simulink model "quadcopter"  (R2023a)
settings: Solver=VariableStepAuto  StartTime=0.0  StopTime=inf  RelTol=1e-3
libraries: slpidlib x4, simulink x1, vrlib x1
settings Model: Creator=sait karadeniz  LastModifiedBy=sait karadeniz
settings DataIOCC: ReturnWorkspaceOutputs=off

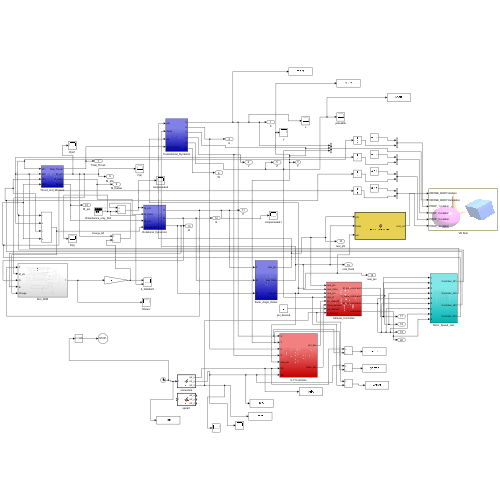
[thumbnail: Simulink's stored preview of the top-level diagram]
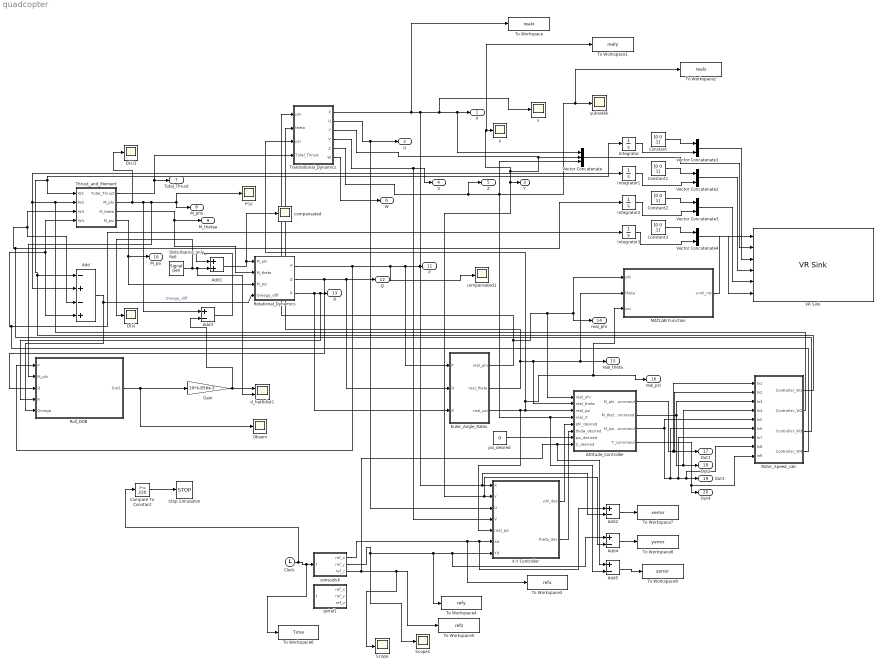
== system quadcopter ==
  Add : Sum  Inputs=-+-+
  Add1 : Sum
  Add{2..5} (4 alike) : Sum  Inputs=+-
  Attitude_Controller : Subsystem
  Clock : Clock
  Compare To Constant : simulink/Logic and Bit Operations/Compare To Constant  relop=>=  const=220  OutDataTypeStr=boolean
  Constant{,1..3} (4 alike) : Constant  Value=[0 0 1]  OutMax=[3]
  D(s) : Scope
  D(s)1 : Scope
  "Disturbance_only_Roll " : SignalGenerator  Amplitude=0.0  Frequency=2  Units=rad/sec
  Euler_Angle_Rates : Subsystem
  F(s) : Scope
  Gain : Gain  Gain=10*4.856e-3
  Integrator{,1..3} (4 alike) : Integrator
  MATLAB Function : MATLAB Function  TreatAsAtomicUnit=on
  Observ : Scope
  Roll_DOB : Subsystem
  Rotational_Dynamics : Subsystem
  Rotor_Speed_calc : Subsystem
  Scope : Scope
  Scope1 : Scope
  Stop Simulation : Stop
  Thrust_and_Moment : Subsystem
  To Workspace : ToWorkspace  VariableName=realx  SampleTime=-1
  To Workspace1 : ToWorkspace  VariableName=realy  SampleTime=-1
  To Workspace2 : ToWorkspace  VariableName=realz  SampleTime=-1
  To Workspace3 : ToWorkspace  VariableName=refx  SampleTime=-1
  To Workspace4 : ToWorkspace  VariableName=refy  SampleTime=-1
  To Workspace5 : ToWorkspace  VariableName=refz  SampleTime=-1
  To Workspace6 : ToWorkspace  VariableName=Time  SampleTime=-1
  To Workspace7 : ToWorkspace  VariableName=xerror  SampleTime=-1
  To Workspace8 : ToWorkspace  VariableName=yerror  SampleTime=-1
  To Workspace9 : ToWorkspace  VariableName=zerror  SampleTime=-1
  Translational_Dynamics : Subsystem
  VR Sink : vrlib/VR Sink  InstantiateOnLoad=on  SampleTime=0.1  ViewEnable=on  RemoteChange=off  RemoteView=off  FieldsWritten=DRONE_BODY.rotation.4.1.1.double#DRONE_BODY.translation.3.1.1.double#PROP_1.rotation.4.1.1.double#PROP_2.rotation.4.1.1.double#PROP_3.rotation.4.1.1.double#PROP_4.rotation.4.1.1.double  WorldFileName=C:\Documents\quadcopter.wrl  WorldDescription=Quadcopter World  AutoView=on  VideoDimensions=[]  AllowVariableSize=off
  Vector Concatenate : Concatenate  NumInputs=3
  Vector Concatenate{1..4} (4 alike) : Concatenate
  X-Y Controller : Subsystem
  compansated : Scope
  compansated1 : Scope
  d_hat6dist1 : Scope  NumInputPorts=2
  psi_desired : Constant  Value=0
  sonsuzluk : MATLAB Function  TreatAsAtomicUnit=on
  spiral1 : MATLAB Function  TreatAsAtomicUnit=on
  x : Scope
  y : Scope
  yükseklik : Scope
  X : Outport
  U : Outport  Port=2
  Y : Outport  Port=3
  V : Outport  Port=4
  Z : Outport  Port=5
  W : Outport  Port=6
  Total_Thrust : Outport  Port=7
  M_phii : Outport  Port=8
  M_thetaa : Outport  Port=9
  M_psi : Outport  Port=10
  P : Outport  Port=11
  Q : Outport  Port=12
  R : Outport  Port=13
  real_phi : Outport  Port=14
  real_theta : Outport  Port=15
  real_psi : Outport  Port=16
  Out1 : Outport  Port=17
  Out2 : Outport  Port=18
  Out3 : Outport  Port=19
  Out4 : Outport  Port=20
  wires:
  Thrust_and_Moment/1(Total_Thrust) -> Translational_Dynamics/4(Total_Thrust), Total_Thrust/1
  Thrust_and_Moment/2(M_phi) -> D(s)1/1, F(s)/1, M_phii/1, Roll_DOB/2(M_phi), Add3/1
  Thrust_and_Moment/3(M_theta) -> Rotational_Dynamics/2(M_theta), M_thetaa/1
  Euler_Angle_Rates/1(real_phi) -> Translational_Dynamics/1(phi), Attitude_Controller/1(real_phi), MATLAB Function/1(phi), real_phi/1
  Euler_Angle_Rates/3(real_psi) -> Attitude_Controller/3(real_psi), Translational_Dynamics/3(psi), real_psi/1, MATLAB Function/3(psi), X-Y Controller/5(real_psi)
  Translational_Dynamics/1(X) -> To Workspace/1, x/1, Vector Concatenate/1, X/1, Add2/2, X-Y Controller/1(X)
  Translational_Dynamics/2(U) -> X-Y Controller/3(U), U/1
  Translational_Dynamics/3(Y) -> Add4/2, X-Y Controller/2(Y), Y/1, To Workspace1/1, y/1, Vector Concatenate/2
  Translational_Dynamics/4(V) -> X-Y Controller/4(V), V/1
  Translational_Dynamics/5(Z) -> To Workspace2/1, yükseklik/1, Add5/2, Attitude_Controller/4(real_Z), Vector Concatenate/3, Z/1
  Translational_Dynamics/6(W) -> W/1
  Add/1 -> Roll_DOB/5(Omega), Rotational_Dynamics/4(Omega_diff)  "Omega_diff"
  Rotational_Dynamics/2(Q) -> Euler_Angle_Rates/2(Q), Q/1, Roll_DOB/3(Q)
  Rotational_Dynamics/3(R) -> Euler_Angle_Rates/3(R), Roll_DOB/4(R), R/1
  Rotational_Dynamics/1(P) -> Roll_DOB/1(P), compansated1/1, Euler_Angle_Rates/1(P), P/1
  Rotor_Speed_calc/1(Controller_W1) -> Integrator/1, Thrust_and_Moment/1(W1), Add/1
  Rotor_Speed_calc/2(Controller_W2) -> Add/2, Integrator1/1, Thrust_and_Moment/2(W2)
  Rotor_Speed_calc/3(Controller_W3) -> Thrust_and_Moment/3(W3), Add/3, Integrator2/1
  Rotor_Speed_calc/4(Controller_W4) -> Add/4, Thrust_and_Moment/4(W4), Integrator3/1
  Vector Concatenate/1 -> VR Sink/2
  MATLAB Function/1(vrml_rot) -> VR Sink/1
  Constant/1 -> Vector Concatenate1/1
  Integrator/1 -> Vector Concatenate1/2
  Constant1/1 -> Vector Concatenate2/1
  Integrator1/1 -> Vector Concatenate2/2
  Constant2/1 -> Vector Concatenate3/1
  Integrator2/1 -> Vector Concatenate3/2
  Constant3/1 -> Vector Concatenate4/1
  Integrator3/1 -> Vector Concatenate4/2
  Vector Concatenate1/1 -> VR Sink/3
  Vector Concatenate2/1 -> VR Sink/4
  Vector Concatenate3/1 -> VR Sink/5
  Vector Concatenate4/1 -> VR Sink/6
  Euler_Angle_Rates/2(real_theta) -> Translational_Dynamics/2(theta), Attitude_Controller/2(real_theta), MATLAB Function/2(theta), real_theta/1
  Attitude_Controller/1(M_phi_command) -> Rotor_Speed_calc/1(In1), Rotor_Speed_calc/2(In2), Out1/1
  Attitude_Controller/2(M_theta_command) -> Rotor_Speed_calc/4(In4), Out2/1, Rotor_Speed_calc/3(In3)
  Attitude_Controller/3(M_psi_command) -> Rotor_Speed_calc/6(In6), Rotor_Speed_calc/7(In7), Rotor_Speed_calc/8(In8), Out3/1, Rotor_Speed_calc/5(In5)
  Attitude_Controller/4(T_command) -> Out4/1, Rotor_Speed_calc/9(In9)
  Add1/1 -> compansated/1, Rotational_Dynamics/1(M_phi)
  Thrust_and_Moment/4(M_psi) -> Rotational_Dynamics/3(M_psi), M_psi/1
  psi_desired/1 -> Attitude_Controller/7(psi_desired)
  X-Y Controller/1(phi_des) -> Attitude_Controller/5(phi_desired)
  X-Y Controller/2(theta_des) -> Attitude_Controller/6(theta_desired)
  Add3/1 -> Add1/1
  "Disturbance_only_Roll "/1 -> D(s)/1, d_hat6dist1/2, Add1/2
  Roll_DOB/1(Out1) -> Gain/1, Observ/1
  Gain/1 -> Add3/2, d_hat6dist1/1
  Clock/1 -> Compare To Constant/1, To Workspace6/1, sonsuzluk/1(t)
  sonsuzluk/1(ref_x) -> To Workspace3/1, Add2/1, X-Y Controller/6(Xd)
  sonsuzluk/3(ref_z) -> Scope/1, To Workspace5/1, Add5/1, Attitude_Controller/8(Z_desired)
  sonsuzluk/2(ref_y) -> Scope1/1, Add4/1, X-Y Controller/7(Yd), To Workspace4/1
  Compare To Constant/1 -> Stop Simulation/1
  Add2/1 -> To Workspace7/1
  Add4/1 -> To Workspace8/1
  Add5/1 -> To Workspace9/1

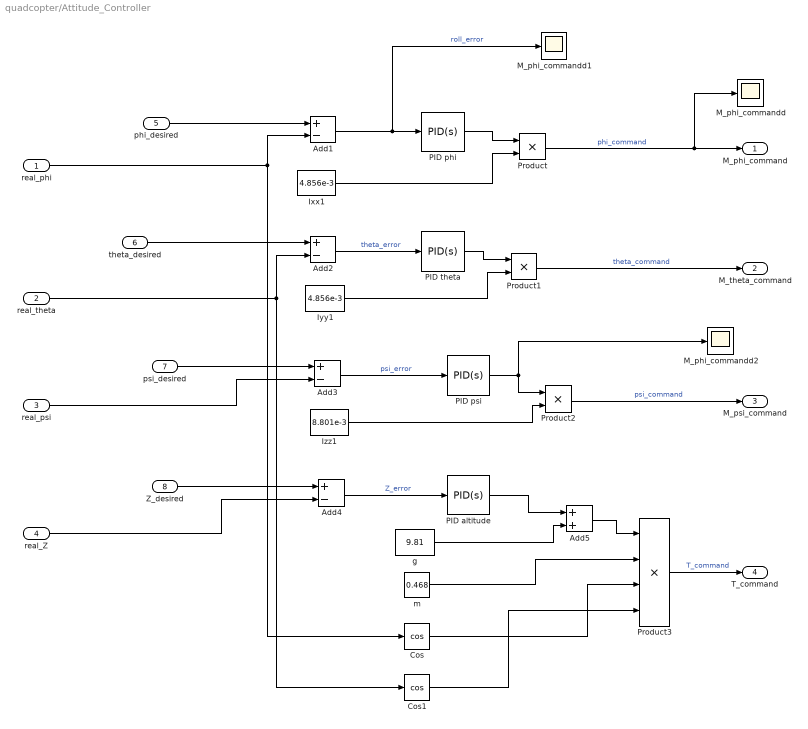
== system quadcopter/Attitude_Controller ==
  real_phi : Inport
  real_theta : Inport  Port=2
  real_psi : Inport  Port=3
  real_Z : Inport  Port=4
  phi_desired : Inport  Port=5
  theta_desired : Inport  Port=6
  psi_desired : Inport  Port=7
  Z_desired : Inport  Port=8
  Add{1..4} (4 alike) : Sum  Inputs=+-
  Add5 : Sum
  Cos : Trigonometry  Operator=cos
  Cos1 : Trigonometry  Operator=cos
  Ixx1 : Constant  Value=4.856e-3
  Iyy1 : Constant  Value=4.856e-3
  Izz1 : Constant  Value=8.801e-3
  M_phi_commandd : Scope
  M_phi_commandd1 : Scope
  M_phi_commandd2 : Scope
  PID altitude : slpidlib/PID Controller  Controller=PID  Form=Parallel  TimeDomain=Continuous-time  UseExternalTs=off  SampleTime=-1  IntegratorMethod=Forward Euler  FilterMethod=Forward Euler  ControllerParametersSource=internal  P=0.3437  I=0.0034  UseKiTs=off  D=0.5550  N=100  UseFilter=on  TunerSelectOption=Transfer Function Based (PID Tuner App)  InitialConditionSource=internal  InitialConditionForIntegrator=0  InitialConditionForFilter=0  DifferentiatorICPrevScaledInput=0  ExternalReset=none  TrackingMode=off  Kt=1  LimitOutput=off  SatLimitsSource=internal  UpperSaturationLimit=inf  LowerSaturationLimit=-inf  LinearizeAsGain=on  AntiWindupMode=none  Kb=1  LimitIntegrator=off  UpperIntegratorSaturationLimit=inf  LowerIntegratorSaturationLimit=-inf  POutMin=[]  POutMax=[]  IOutMin=[]  IOutMax=[]  DOutMin=[]  DOutMax=[]  NOutMin=[]  NOutMax=[]  SumOutMin=[]  SumOutMax=[]  SaturationOutMin=[]  SaturationOutMax=[]  PParamMin=[]  PParamMax=[]  IParamMin=[]  IParamMax=[]  DParamMin=[]  DParamMax=[]  NParamMin=[]  NParamMax=[]  KbParamMin=[]  KbParamMax=[]  KtParamMin=[]  KtParamMax=[]  KbOutMin=[]  KbOutMax=[]  KtOutMin=[]  KtOutMax=[]  IntegratorOutMin=[]  IntegratorOutMax=[]  FilterOutMin=[]  FilterOutMax=[]  SumI1OutMin=[]  SumI1OutMax=[]  SumI2OutMin=[]  SumI2OutMax=[]  SumI3OutMin=[]  SumI3OutMax=[]  SumI4OutMin=[]  SumI4OutMax=[]  SumDOutMin=[]  SumDOutMax=[]  DifferentiatorOutMin=[]  DifferentiatorOutMax=[]  FilterDiffOutCoefMin=[]  FilterDiffOutCoefMax=[]  ReciprocalOutMin=[]  ReciprocalOutMax=[]  SumDenOutMin=[]  SumDenOutMax=[]  SumNumOutMin=[]  SumNumOutMax=[]  DivideOutMin=[]  DivideOutMax=[]  UdiffTsProdOutMin=[]  UdiffTsProdOutMax=[]  NTsProdOutMin=[]  NTsProdOutMax=[]  UintegralTsProdOutMin=[]  UintegralTsProdOutMax=[]  UngainTsProdOutMin=[]  UngainTsProdOutMax=[]  ClampingZeroOutDataTypeStr=Inherit: Inherit via back propagation  ClampingZeroOutMin=[]  ClampingZeroOutMax=[]  FilterDenConstantOutDataTypeStr=Inherit: Inherit via back propagation  FilterDenConstantOutMin=[]  FilterDenConstantOutMax=[]  PCopyOutDataTypeStr=Inherit: Inherit via back propagation  PCopyOutMin=[]  PCopyOutMax=[]  NCopyOutDataTypeStr=Inherit: Inherit via back propagation  NCopyOutMin=[]  NCopyOutMax=[]  IntegratorContinuousStateAttributes=''  IntegratorStateMustResolveToSignalObject=off  IntegratorRTWStateStorageClass=Auto  FilterContinuousStateAttributes=''  FilterStateMustResolveToSignalObject=off  FilterRTWStateStorageClass=Auto  ParallelPVariant=InternalParameters  IdealPVariant=Disabled  IVariant=InternalParameters  DVariant=InternalParameters  IntegratorVariant=Continuous  SatVariant=Disabled  AWVariant=Passthrough  PCopyVariant=Disabled  TRVariant=Disabled  FdbkBlocksVariant=Forward  IdealPFdbkVariant=Disabled  SatFdbkVariant=Disabled  DerivativeFilterVariant=ContFilter  NVariant=InternalParameters  NCopyVariant=Disabled  FilterICVariant=InternalICsFilter  IntegratorICVariant=InternalICs  ExternalResetVariant=Disabled  TRSumVariant=Passthrough  SumFdbkVariant=Disabled  SumVariant=Sum_PID  TsampFilterVariant=InternalTs  TsampNgainVariant=Passthrough  TsampIntegralVariant=Disabled_SignalSpec  ExternalSaturationOutDataTypeStr=Inherit: Same as second input
  PID phi : slpidlib/PID Controller  Controller=PID  Form=Parallel  TimeDomain=Continuous-time  UseExternalTs=off  SampleTime=-1  IntegratorMethod=Forward Euler  FilterMethod=Forward Euler  ControllerParametersSource=internal  P=6  I=1.5  UseKiTs=off  D=2  N=20  UseFilter=on  TunerSelectOption=Transfer Function Based (PID Tuner App)  InitialConditionSource=internal  InitialConditionForIntegrator=0  InitialConditionForFilter=0  DifferentiatorICPrevScaledInput=0  ExternalReset=none  TrackingMode=off  Kt=1  LimitOutput=off  SatLimitsSource=internal  UpperSaturationLimit=inf  LowerSaturationLimit=-inf  LinearizeAsGain=on  AntiWindupMode=none  Kb=1  LimitIntegrator=off  UpperIntegratorSaturationLimit=inf  LowerIntegratorSaturationLimit=-inf  POutMin=[]  POutMax=[]  IOutMin=[]  IOutMax=[]  DOutMin=[]  DOutMax=[]  NOutMin=[]  NOutMax=[]  SumOutMin=[]  SumOutMax=[]  SaturationOutMin=[]  SaturationOutMax=[]  PParamMin=[]  PParamMax=[]  IParamMin=[]  IParamMax=[]  DParamMin=[]  DParamMax=[]  NParamMin=[]  NParamMax=[]  KbParamMin=[]  KbParamMax=[]  KtParamMin=[]  KtParamMax=[]  KbOutMin=[]  KbOutMax=[]  KtOutMin=[]  KtOutMax=[]  IntegratorOutMin=[]  IntegratorOutMax=[]  FilterOutMin=[]  FilterOutMax=[]  SumI1OutMin=[]  SumI1OutMax=[]  SumI2OutMin=[]  SumI2OutMax=[]  SumI3OutMin=[]  SumI3OutMax=[]  SumI4OutMin=[]  SumI4OutMax=[]  SumDOutMin=[]  SumDOutMax=[]  DifferentiatorOutMin=[]  DifferentiatorOutMax=[]  FilterDiffOutCoefMin=[]  FilterDiffOutCoefMax=[]  ReciprocalOutMin=[]  ReciprocalOutMax=[]  SumDenOutMin=[]  SumDenOutMax=[]  SumNumOutMin=[]  SumNumOutMax=[]  DivideOutMin=[]  DivideOutMax=[]  UdiffTsProdOutMin=[]  UdiffTsProdOutMax=[]  NTsProdOutMin=[]  NTsProdOutMax=[]  UintegralTsProdOutMin=[]  UintegralTsProdOutMax=[]  UngainTsProdOutMin=[]  UngainTsProdOutMax=[]  ClampingZeroOutDataTypeStr=Inherit: Inherit via back propagation  ClampingZeroOutMin=[]  ClampingZeroOutMax=[]  FilterDenConstantOutDataTypeStr=Inherit: Inherit via back propagation  FilterDenConstantOutMin=[]  FilterDenConstantOutMax=[]  PCopyOutDataTypeStr=Inherit: Inherit via back propagation  PCopyOutMin=[]  PCopyOutMax=[]  NCopyOutDataTypeStr=Inherit: Inherit via back propagation  NCopyOutMin=[]  NCopyOutMax=[]  IntegratorContinuousStateAttributes=''  IntegratorStateMustResolveToSignalObject=off  IntegratorRTWStateStorageClass=Auto  FilterContinuousStateAttributes=''  FilterStateMustResolveToSignalObject=off  FilterRTWStateStorageClass=Auto  ParallelPVariant=InternalParameters  IdealPVariant=Disabled  IVariant=InternalParameters  DVariant=InternalParameters  IntegratorVariant=Continuous  SatVariant=Disabled  AWVariant=Passthrough  PCopyVariant=Disabled  TRVariant=Disabled  FdbkBlocksVariant=Forward  IdealPFdbkVariant=Disabled  SatFdbkVariant=Disabled  DerivativeFilterVariant=ContFilter  NVariant=InternalParameters  NCopyVariant=Disabled  FilterICVariant=InternalICsFilter  IntegratorICVariant=InternalICs  ExternalResetVariant=Disabled  TRSumVariant=Passthrough  SumFdbkVariant=Disabled  SumVariant=Sum_PID  TsampFilterVariant=InternalTs  TsampNgainVariant=Passthrough  TsampIntegralVariant=Disabled_SignalSpec  ExternalSaturationOutDataTypeStr=Inherit: Same as second input
  PID psi : slpidlib/PID Controller  Controller=PID  Form=Parallel  TimeDomain=Continuous-time  UseExternalTs=off  SampleTime=-1  IntegratorMethod=Forward Euler  FilterMethod=Forward Euler  ControllerParametersSource=internal  P=0.3  I=0.001  UseKiTs=off  D=0.7  N=100  UseFilter=on  TunerSelectOption=Transfer Function Based (PID Tuner App)  InitialConditionSource=internal  InitialConditionForIntegrator=0  InitialConditionForFilter=0  DifferentiatorICPrevScaledInput=0  ExternalReset=none  TrackingMode=off  Kt=1  LimitOutput=off  SatLimitsSource=internal  UpperSaturationLimit=inf  LowerSaturationLimit=-inf  LinearizeAsGain=on  AntiWindupMode=none  Kb=1  LimitIntegrator=on  UpperIntegratorSaturationLimit=0.5  LowerIntegratorSaturationLimit=-0.5  POutMin=[]  POutMax=[]  IOutMin=[]  IOutMax=[]  DOutMin=[]  DOutMax=[]  NOutMin=[]  NOutMax=[]  SumOutMin=[]  SumOutMax=[]  SaturationOutMin=[]  SaturationOutMax=[]  PParamMin=[]  PParamMax=[]  IParamMin=[]  IParamMax=[]  DParamMin=[]  DParamMax=[]  NParamMin=[]  NParamMax=[]  KbParamMin=[]  KbParamMax=[]  KtParamMin=[]  KtParamMax=[]  KbOutMin=[]  KbOutMax=[]  KtOutMin=[]  KtOutMax=[]  IntegratorOutMin=[]  IntegratorOutMax=[]  FilterOutMin=[]  FilterOutMax=[]  SumI1OutMin=[]  SumI1OutMax=[]  SumI2OutMin=[]  SumI2OutMax=[]  SumI3OutMin=[]  SumI3OutMax=[]  SumI4OutMin=[]  SumI4OutMax=[]  SumDOutMin=[]  SumDOutMax=[]  DifferentiatorOutMin=[]  DifferentiatorOutMax=[]  FilterDiffOutCoefMin=[]  FilterDiffOutCoefMax=[]  ReciprocalOutMin=[]  ReciprocalOutMax=[]  SumDenOutMin=[]  SumDenOutMax=[]  SumNumOutMin=[]  SumNumOutMax=[]  DivideOutMin=[]  DivideOutMax=[]  UdiffTsProdOutMin=[]  UdiffTsProdOutMax=[]  NTsProdOutMin=[]  NTsProdOutMax=[]  UintegralTsProdOutMin=[]  UintegralTsProdOutMax=[]  UngainTsProdOutMin=[]  UngainTsProdOutMax=[]  ClampingZeroOutDataTypeStr=Inherit: Inherit via back propagation  ClampingZeroOutMin=[]  ClampingZeroOutMax=[]  FilterDenConstantOutDataTypeStr=Inherit: Inherit via back propagation  FilterDenConstantOutMin=[]  FilterDenConstantOutMax=[]  PCopyOutDataTypeStr=Inherit: Inherit via back propagation  PCopyOutMin=[]  PCopyOutMax=[]  NCopyOutDataTypeStr=Inherit: Inherit via back propagation  NCopyOutMin=[]  NCopyOutMax=[]  IntegratorContinuousStateAttributes=''  IntegratorStateMustResolveToSignalObject=off  IntegratorRTWStateStorageClass=Auto  FilterContinuousStateAttributes=''  FilterStateMustResolveToSignalObject=off  FilterRTWStateStorageClass=Auto  ParallelPVariant=InternalParameters  IdealPVariant=Disabled  IVariant=InternalParameters  DVariant=InternalParameters  IntegratorVariant=Continuous  SatVariant=Disabled  AWVariant=Passthrough  PCopyVariant=Disabled  TRVariant=Disabled  FdbkBlocksVariant=Forward  IdealPFdbkVariant=Disabled  SatFdbkVariant=Disabled  DerivativeFilterVariant=ContFilter  NVariant=InternalParameters  NCopyVariant=Disabled  FilterICVariant=InternalICsFilter  IntegratorICVariant=InternalICs  ExternalResetVariant=Disabled  TRSumVariant=Passthrough  SumFdbkVariant=Disabled  SumVariant=Sum_PID  TsampFilterVariant=InternalTs  TsampNgainVariant=Passthrough  TsampIntegralVariant=Disabled_SignalSpec  ExternalSaturationOutDataTypeStr=Inherit: Same as second input
  PID theta : slpidlib/PID Controller  Controller=PID  Form=Parallel  TimeDomain=Continuous-time  UseExternalTs=off  SampleTime=-1  IntegratorMethod=Forward Euler  FilterMethod=Forward Euler  ControllerParametersSource=internal  P=5  I=3  UseKiTs=off  D=3  N=100  UseFilter=on  TunerSelectOption=Transfer Function Based (PID Tuner App)  InitialConditionSource=internal  InitialConditionForIntegrator=0  InitialConditionForFilter=0  DifferentiatorICPrevScaledInput=0  ExternalReset=none  TrackingMode=off  Kt=1  LimitOutput=off  SatLimitsSource=internal  UpperSaturationLimit=inf  LowerSaturationLimit=-inf  LinearizeAsGain=on  AntiWindupMode=none  Kb=1  LimitIntegrator=off  UpperIntegratorSaturationLimit=inf  LowerIntegratorSaturationLimit=-inf  POutMin=[]  POutMax=[]  IOutMin=[]  IOutMax=[]  DOutMin=[]  DOutMax=[]  NOutMin=[]  NOutMax=[]  SumOutMin=[]  SumOutMax=[]  SaturationOutMin=[]  SaturationOutMax=[]  PParamMin=[]  PParamMax=[]  IParamMin=[]  IParamMax=[]  DParamMin=[]  DParamMax=[]  NParamMin=[]  NParamMax=[]  KbParamMin=[]  KbParamMax=[]  KtParamMin=[]  KtParamMax=[]  KbOutMin=[]  KbOutMax=[]  KtOutMin=[]  KtOutMax=[]  IntegratorOutMin=[]  IntegratorOutMax=[]  FilterOutMin=[]  FilterOutMax=[]  SumI1OutMin=[]  SumI1OutMax=[]  SumI2OutMin=[]  SumI2OutMax=[]  SumI3OutMin=[]  SumI3OutMax=[]  SumI4OutMin=[]  SumI4OutMax=[]  SumDOutMin=[]  SumDOutMax=[]  DifferentiatorOutMin=[]  DifferentiatorOutMax=[]  FilterDiffOutCoefMin=[]  FilterDiffOutCoefMax=[]  ReciprocalOutMin=[]  ReciprocalOutMax=[]  SumDenOutMin=[]  SumDenOutMax=[]  SumNumOutMin=[]  SumNumOutMax=[]  DivideOutMin=[]  DivideOutMax=[]  UdiffTsProdOutMin=[]  UdiffTsProdOutMax=[]  NTsProdOutMin=[]  NTsProdOutMax=[]  UintegralTsProdOutMin=[]  UintegralTsProdOutMax=[]  UngainTsProdOutMin=[]  UngainTsProdOutMax=[]  ClampingZeroOutDataTypeStr=Inherit: Inherit via back propagation  ClampingZeroOutMin=[]  ClampingZeroOutMax=[]  FilterDenConstantOutDataTypeStr=Inherit: Inherit via back propagation  FilterDenConstantOutMin=[]  FilterDenConstantOutMax=[]  PCopyOutDataTypeStr=Inherit: Inherit via back propagation  PCopyOutMin=[]  PCopyOutMax=[]  NCopyOutDataTypeStr=Inherit: Inherit via back propagation  NCopyOutMin=[]  NCopyOutMax=[]  IntegratorContinuousStateAttributes=''  IntegratorStateMustResolveToSignalObject=off  IntegratorRTWStateStorageClass=Auto  FilterContinuousStateAttributes=''  FilterStateMustResolveToSignalObject=off  FilterRTWStateStorageClass=Auto  ParallelPVariant=InternalParameters  IdealPVariant=Disabled  IVariant=InternalParameters  DVariant=InternalParameters  IntegratorVariant=Continuous  SatVariant=Disabled  AWVariant=Passthrough  PCopyVariant=Disabled  TRVariant=Disabled  FdbkBlocksVariant=Forward  IdealPFdbkVariant=Disabled  SatFdbkVariant=Disabled  DerivativeFilterVariant=ContFilter  NVariant=InternalParameters  NCopyVariant=Disabled  FilterICVariant=InternalICsFilter  IntegratorICVariant=InternalICs  ExternalResetVariant=Disabled  TRSumVariant=Passthrough  SumFdbkVariant=Disabled  SumVariant=Sum_PID  TsampFilterVariant=InternalTs  TsampNgainVariant=Passthrough  TsampIntegralVariant=Disabled_SignalSpec  ExternalSaturationOutDataTypeStr=Inherit: Same as second input
  Product : Product
  Product1 : Product
  Product2 : Product
  Product3 : Product  Inputs=4
  g : Constant  Value=9.81
  m : Constant  Value=0.468
  M_phi_command : Outport
  M_theta_command : Outport  Port=2
  M_psi_command : Outport  Port=3
  T_command : Outport  Port=4
  wires:
  phi_desired/1 -> Add1/1
  Cos/1 -> Product3/3
  Cos1/1 -> Product3/4
  real_phi/1 -> Add1/2, Cos/1
  Izz1/1 -> Product2/2
  PID altitude/1 -> Add5/1
  Add1/1 -> M_phi_commandd1/1, PID phi/1  "roll_error"
  real_Z/1 -> Add4/2
  Add3/1 -> PID psi/1  "psi_error"
  PID theta/1 -> Product1/1
  Iyy1/1 -> Product1/2
  Ixx1/1 -> Product/2
  theta_desired/1 -> Add2/1
  m/1 -> Product3/2
  Product3/1 -> T_command/1  "T_command"
  Product1/1 -> M_theta_command/1  "theta_command"
  Add5/1 -> Product3/1
  psi_desired/1 -> Add3/1
  real_psi/1 -> Add3/2
  Add2/1 -> PID theta/1  "theta_error"
  Z_desired/1 -> Add4/1
  Add4/1 -> PID altitude/1  "Z_error"
  Product/1 -> M_phi_commandd/1, M_phi_command/1  "phi_command"
  real_theta/1 -> Add2/2, Cos1/1
  Product2/1 -> M_psi_command/1  "psi_command"
  PID psi/1 -> M_phi_commandd2/1, Product2/1
  g/1 -> Add5/2
  PID phi/1 -> Product/1

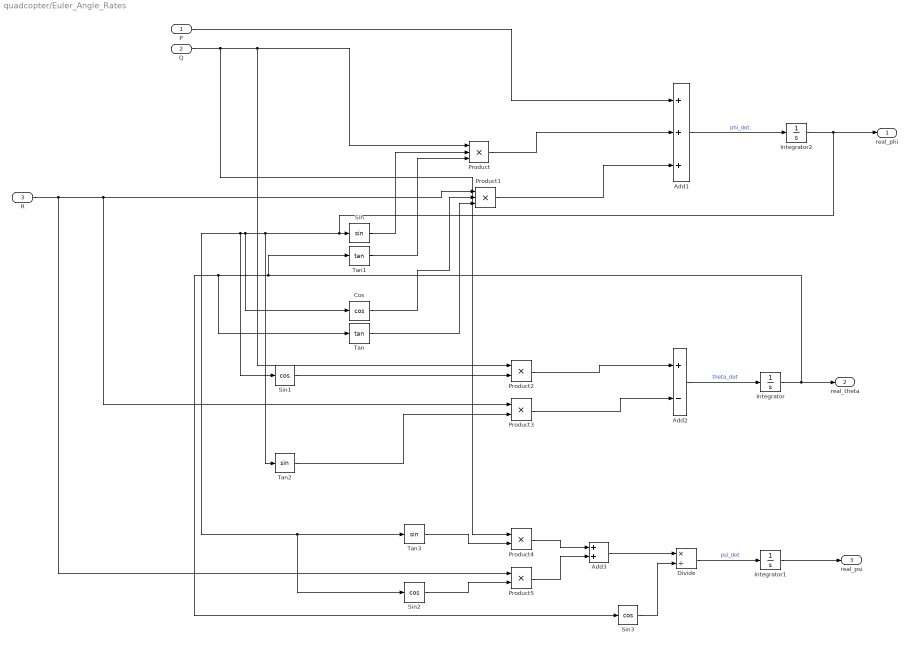
== system quadcopter/Euler_Angle_Rates ==
  P : Inport
  Q : Inport  Port=2
  R : Inport  Port=3
  Add1 : Sum  Inputs=+++
  Add2 : Sum  Inputs=+-
  Add3 : Sum
  Cos : Trigonometry  Operator=cos
  Divide : Product  Inputs=*/
  Integrator : Integrator
  Integrator1 : Integrator
  Integrator2 : Integrator
  Product : Product  Inputs=3
  Product1 : Product  Inputs=3
  Product{2..5} (4 alike) : Product
  Sin : Trigonometry
  Sin1 : Trigonometry  Operator=cos
  Sin2 : Trigonometry  Operator=cos
  Sin3 : Trigonometry  Operator=cos
  Tan : Trigonometry  Operator=tan
  Tan1 : Trigonometry  Operator=tan
  Tan2 : Trigonometry
  Tan3 : Trigonometry
  real_phi : Outport
  real_theta : Outport  Port=2
  real_psi : Outport  Port=3
  wires:
  Tan1/1 -> Product/3
  Integrator2/1 -> real_phi/1, Sin2/1, Tan3/1, Sin1/1, Cos/1, Tan2/1, Sin/1
  Add1/1 -> Integrator2/1  "phi_dot"
  Divide/1 -> Integrator1/1  "psi_dot"
  Product3/1 -> Add2/2
  Integrator/1 -> real_theta/1, Sin3/1, Tan/1, Tan1/1
  Product1/1 -> Add1/3
  Tan3/1 -> Product4/2
  Sin2/1 -> Product5/2
  Tan2/1 -> Product3/2
  Integrator1/1 -> real_psi/1
  Product2/1 -> Add2/1
  Cos/1 -> Product1/2
  Add2/1 -> Integrator/1  "theta_dot"
  Product4/1 -> Add3/1
  Sin/1 -> Product/2
  Tan/1 -> Product1/3
  Add3/1 -> Divide/1
  Product/1 -> Add1/2
  Sin1/1 -> Product2/2
  Product5/1 -> Add3/2
  Sin3/1 -> Divide/2
  Q/1 -> Product4/1, Product/1, Product2/1
  R/1 -> Product5/1, Product3/1, Product1/1
  P/1 -> Add1/1

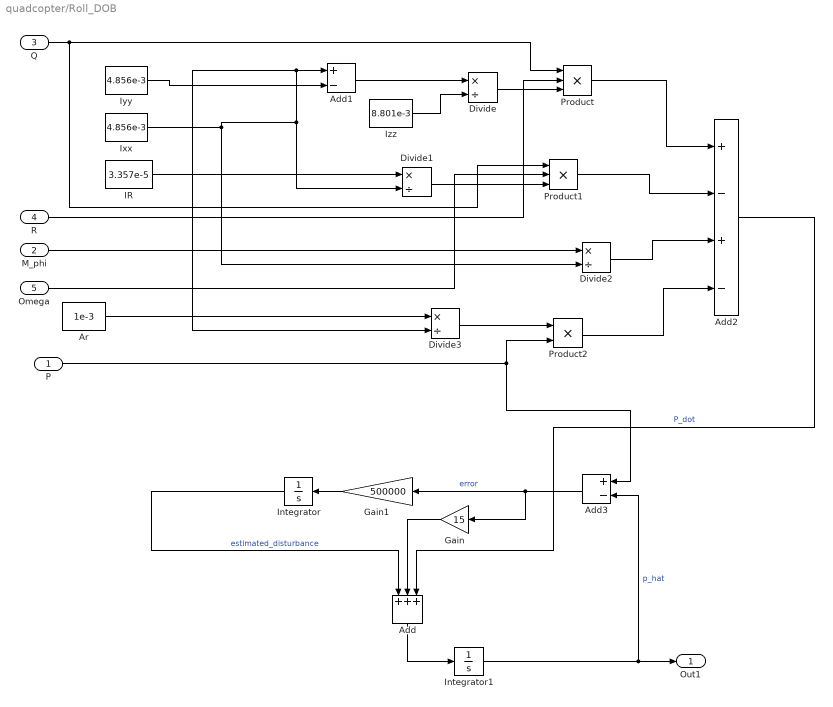
== system quadcopter/Roll_DOB ==
  P : Inport
  M_phi : Inport  Port=2
  Q : Inport  Port=3
  R : Inport  Port=4
  Omega : Inport  Port=5
  Add : Sum  Inputs=+++
  Add1 : Sum  Inputs=+-
  Add2 : Sum  Inputs=+-+-
  Add3 : Sum  Inputs=+-
  Ar : Constant  Value=1e-3
  Divide{,1..3} (4 alike) : Product  Inputs=*/
  Gain : Gain  Gain=15
  Gain1 : Gain  Gain=500000
  IR : Constant  Value=3.357e-5
  Integrator : Integrator
  Integrator1 : Integrator
  Ixx : Constant  Value=4.856e-3
  Iyy : Constant  Value=4.856e-3
  Izz : Constant  Value=8.801e-3
  Product : Product  Inputs=3
  Product1 : Product  Inputs=3
  Product2 : Product
  Out1 : Outport
  wires:
  Divide/1 -> Product/3
  Divide3/1 -> Product2/1
  Ar/1 -> Divide3/1
  Product1/1 -> Add2/2
  Izz/1 -> Divide/2
  Product/1 -> Add2/1
  Divide2/1 -> Add2/3
  Ixx/1 -> Add1/1, Divide3/2, Divide1/2, Divide2/2
  IR/1 -> Divide1/1
  Divide1/1 -> Product1/3
  M_phi/1 -> Divide2/1
  Add1/1 -> Divide/1
  Product2/1 -> Add2/4
  Iyy/1 -> Add1/2
  Q/1 -> Product1/1, Product/1
  R/1 -> Product/2
  Omega/1 -> Product1/2
  P/1 -> Add3/1, Product2/2
  Add3/1 -> Gain/1, Gain1/1  "error"
  Gain1/1 -> Integrator/1
  Integrator/1 -> Add/1  "estimated_disturbance"
  Add2/1 -> Add/3  "P_dot"
  Gain/1 -> Add/2
  Add/1 -> Integrator1/1
  Integrator1/1 -> Add3/2, Out1/1  "p_hat"

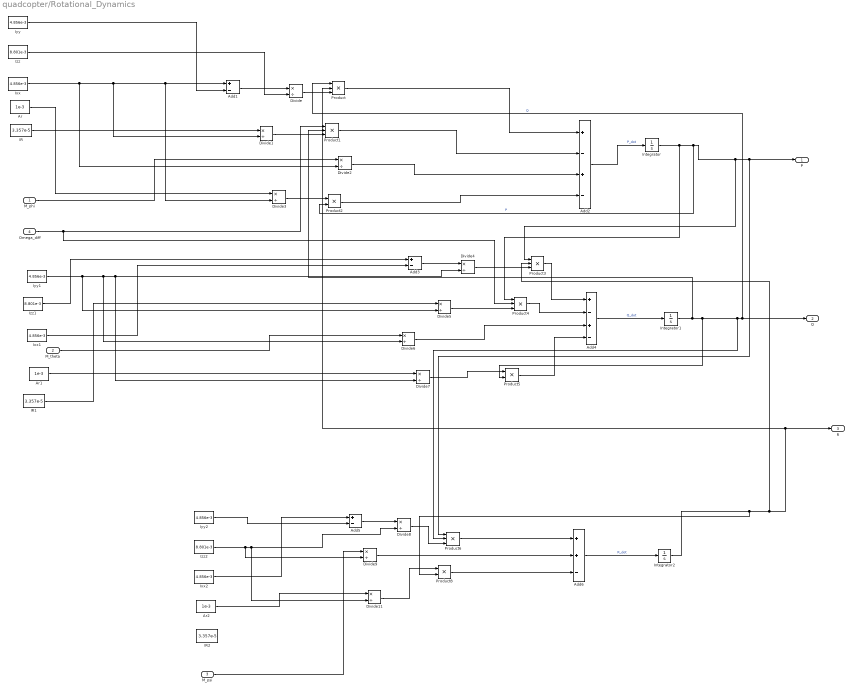
== system quadcopter/Rotational_Dynamics ==
  M_phi : Inport
  M_theta : Inport  Port=2
  M_psi : Inport  Port=3
  Omega_diff : Inport  Port=4
  Add1 : Sum  Inputs=+-
  Add2 : Sum  Inputs=+-+-
  Add3 : Sum  Inputs=+-
  Add4 : Sum  Inputs=+-+-
  Add5 : Sum  Inputs=+-
  Add6 : Sum  Inputs=++-
  Ar : Constant  Value=1e-3
  Ar1 : Constant  Value=1e-3
  Ar2 : Constant  Value=1e-3
  Divide{,1..9,11} (11 alike) : Product  Inputs=*/
  IR : Constant  Value=3.357e-5
  IR1 : Constant  Value=3.357e-5
  IR2 : Constant  Value=3.357e-5
  Integrator : Integrator
  Integrator1 : Integrator
  Integrator2 : Integrator
  Ixx : Constant  Value=4.856e-3
  Ixx1 : Constant  Value=4.856e-3
  Ixx2 : Constant  Value=4.856e-3
  Iyy : Constant  Value=4.856e-3
  Iyy1 : Constant  Value=4.856e-3
  Iyy2 : Constant  Value=4.856e-3
  Izz : Constant  Value=8.801e-3
  Izz1 : Constant  Value=8.801e-3
  Izz2 : Constant  Value=8.801e-3
  Product{,1,3..4,6} (5 alike) : Product  Inputs=3
  Product2 : Product
  Product5 : Product
  Product8 : Product
  P : Outport
  Q : Outport  Port=2
  R : Outport  Port=3
  wires:
  Integrator/1 -> Product4/1, Product2/2, Product3/1, Product6/1, P/1  "P"
  Product6/1 -> Add6/1
  Add6/1 -> Integrator2/1  "R_dot"
  Divide2/1 -> Add2/3
  Add3/1 -> Divide4/1
  Add5/1 -> Divide8/1
  Divide3/1 -> Product2/1
  Integrator1/1 -> Product1/2, Product5/2, Product/1, Q/1, Product6/2  "Q"
  Product/1 -> Add2/1
  Product1/1 -> Add2/2
  Divide11/1 -> Product8/1
  Add1/1 -> Divide/1
  Product5/1 -> Add4/4
  Integrator2/1 -> Product8/2, Product3/2, R/1, Product/2
  Divide8/1 -> Product6/3
  Product3/1 -> Add4/1
  Add2/1 -> Integrator/1  "P_dot"
  Product2/1 -> Add2/4
  Divide5/1 -> Product4/3
  Divide4/1 -> Product3/3
  Divide6/1 -> Add4/3
  Divide7/1 -> Product5/1
  Product4/1 -> Add4/2
  Add4/1 -> Integrator1/1  "Q_dot"
  Divide9/1 -> Add6/2
  Divide/1 -> Product/3
  Divide1/1 -> Product1/3
  Product8/1 -> Add6/3
  Ixx/1 -> Divide2/2, Divide1/2, Divide3/2, Add1/1
  IR/1 -> Divide1/1
  Omega_diff/1 -> Product4/2, Product1/1
  M_phi/1 -> Divide2/1
  Ar/1 -> Divide3/1
  Iyy/1 -> Add1/2
  Izz/1 -> Divide/2
  Izz1/1 -> Add3/1
  Ixx1/1 -> Add3/2
  Iyy1/1 -> Divide5/2, Divide6/2, Divide7/2, Divide4/2
  IR1/1 -> Divide5/1
  M_theta/1 -> Divide6/1
  Ar1/1 -> Divide7/1
  Ixx2/1 -> Add5/1
  Iyy2/1 -> Add5/2
  Izz2/1 -> Divide9/2, Divide11/2, Divide8/2
  M_psi/1 -> Divide9/1
  Ar2/1 -> Divide11/1

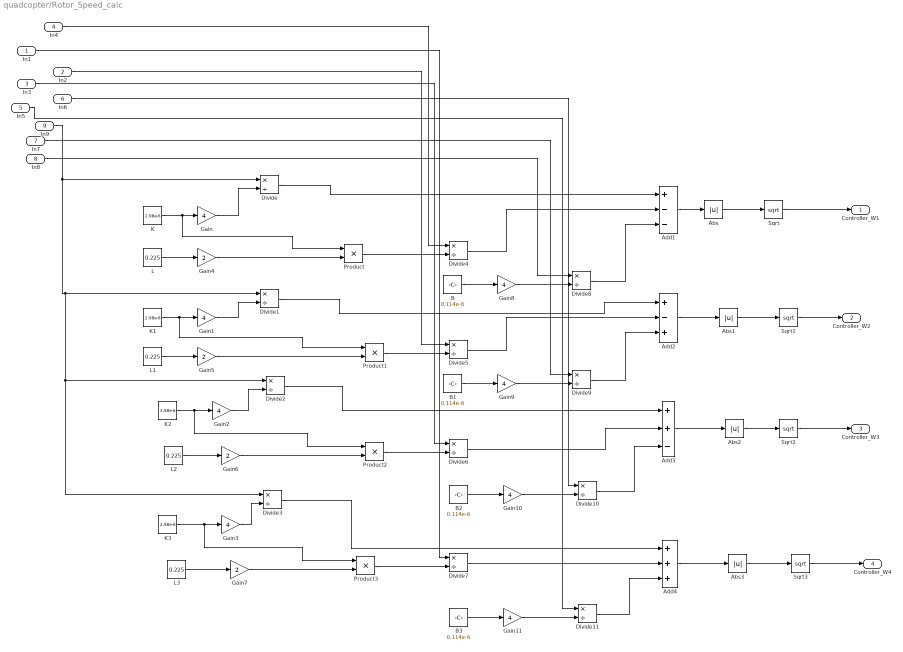
== system quadcopter/Rotor_Speed_calc ==
  In1 : Inport
  In2 : Inport  Port=2
  In3 : Inport  Port=3
  In4 : Inport  Port=4
  In5 : Inport  Port=5
  In6 : Inport  Port=6
  In7 : Inport  Port=7
  In8 : Inport  Port=8
  In9 : Inport  Port=9
  Abs{,1..3} (4 alike) : Abs  SaturateOnIntegerOverflow=off
  Add1 : Sum  Inputs=+--
  Add2 : Sum  Inputs=+-+
  Add3 : Sum  Inputs=++-
  Add4 : Sum  Inputs=+++
  B{,1..3} (4 alike) : Constant  Value=0.114e-6
  Divide{,1..11} (12 alike) : Product  Inputs=*/
  Gain{,1..3,8..11} (8 alike) : Gain  Gain=4
  Gain{4..7} (4 alike) : Gain  Gain=2
  K{,1..3} (4 alike) : Constant  Value=2.98e-6
  L{,1..3} (4 alike) : Constant  Value=0.225
  Product{,1..3} (4 alike) : Product
  Sqrt{,1..3} (4 alike) : Sqrt
  Controller_W1 : Outport
  Controller_W2 : Outport  Port=2
  Controller_W3 : Outport  Port=3
  Controller_W4 : Outport  Port=4
  wires:
  K/1 -> Product/1, Gain/1
  Sqrt1/1 -> Controller_W2/1
  Divide1/1 -> Add2/1
  Divide/1 -> Add1/1
  Gain3/1 -> Divide3/2
  Gain/1 -> Divide/2
  Divide8/1 -> Add1/3
  Add4/1 -> Abs3/1
  B/1 -> Gain8/1
  B2/1 -> Gain10/1
  Gain5/1 -> Product1/2
  Divide9/1 -> Add2/3
  Abs2/1 -> Sqrt2/1
  Add2/1 -> Abs1/1
  Divide5/1 -> Add2/2
  B3/1 -> Gain11/1
  Add3/1 -> Abs2/1
  Divide11/1 -> Add4/3
  Divide10/1 -> Add3/3
  K1/1 -> Product1/1, Gain1/1
  Divide4/1 -> Add1/2
  In9/1 -> Divide3/1, Divide2/1, Divide1/1, Divide/1
  Product3/1 -> Divide7/2
  Product/1 -> Divide4/2
  K2/1 -> Product2/1, Gain2/1
  Divide2/1 -> Add3/1
  Gain1/1 -> Divide1/2
  Divide3/1 -> Add4/1
  Divide7/1 -> Add4/2
  L1/1 -> Gain5/1
  Gain9/1 -> Divide9/2
  Abs3/1 -> Sqrt3/1
  L/1 -> Gain4/1
  Abs1/1 -> Sqrt1/1
  B1/1 -> Gain9/1
  Sqrt/1 -> Controller_W1/1
  Gain4/1 -> Product/2
  L2/1 -> Gain6/1
  In8/1 -> Divide8/1
  In5/1 -> Divide11/1
  Gain6/1 -> Product2/2
  In3/1 -> Divide6/1
  Product1/1 -> Divide5/2
  Product2/1 -> Divide6/2
  In1/1 -> Divide7/1
  Divide6/1 -> Add3/2
  Gain8/1 -> Divide8/2
  L3/1 -> Gain7/1
  Sqrt3/1 -> Controller_W4/1
  K3/1 -> Product3/1, Gain3/1
  Gain10/1 -> Divide10/2
  Gain7/1 -> Product3/2
  Gain11/1 -> Divide11/2
  Gain2/1 -> Divide2/2
  Sqrt2/1 -> Controller_W3/1
  Abs/1 -> Sqrt/1
  Add1/1 -> Abs/1
  In4/1 -> Divide4/1
  In6/1 -> Divide10/1
  In7/1 -> Divide9/1
  In2/1 -> Divide5/1

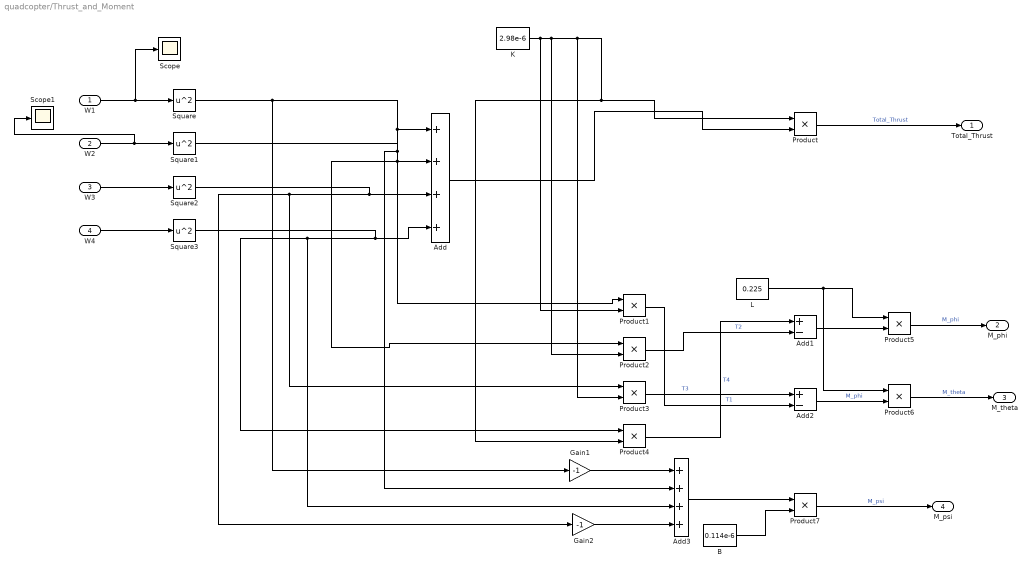
== system quadcopter/Thrust_and_Moment ==
  W1 : Inport
  W2 : Inport  Port=2
  W3 : Inport  Port=3
  W4 : Inport  Port=4
  Add : Sum  Inputs=++++
  Add1 : Sum  Inputs=+-
  Add2 : Sum  Inputs=+-
  Add3 : Sum  Inputs=++++
  B : Constant  Value=0.114e-6
  Gain1 : Gain  Gain=-1
  Gain2 : Gain  Gain=-1
  K : Constant  Value=2.98e-6
  L : Constant  Value=0.225
  Product{,1..7} (8 alike) : Product
  Scope : Scope
  Scope1 : Scope
  Square{,1..3} (4 alike) : Math  Operator=square
  Total_Thrust : Outport
  M_phi : Outport  Port=2
  M_theta : Outport  Port=3
  M_psi : Outport  Port=4
  wires:
  Square1/1 -> Add3/2, Add/2, Product2/1
  Product3/1 -> Add2/1  "T3"
  Product1/1 -> Add2/2  "T1"
  Square3/1 -> Product4/1, Add3/3, Add/4
  Add3/1 -> Product7/1
  Square2/1 -> Gain2/1, Product3/1, Add/3
  Product7/1 -> M_psi/1  "M_psi"
  W1/1 -> Scope/1, Square/1
  K/1 -> Product2/2, Product4/2, Product/1, Product3/2, Product1/2
  W4/1 -> Square3/1
  Product2/1 -> Add1/2  "T2"
  Add1/1 -> Product5/2
  W2/1 -> Scope1/1, Square1/1
  Product5/1 -> M_phi/1  "M_phi"
  Square/1 -> Add/1, Product1/1, Gain1/1
  Product/1 -> Total_Thrust/1  "Total_Thrust"
  Gain2/1 -> Add3/4
  L/1 -> Product6/1, Product5/1
  Add2/1 -> Product6/2  "M_phi"
  W3/1 -> Square2/1
  B/1 -> Product7/2
  Product4/1 -> Add1/1  "T4"
  Add/1 -> Product/2
  Gain1/1 -> Add3/1
  Product6/1 -> M_theta/1  "M_theta"

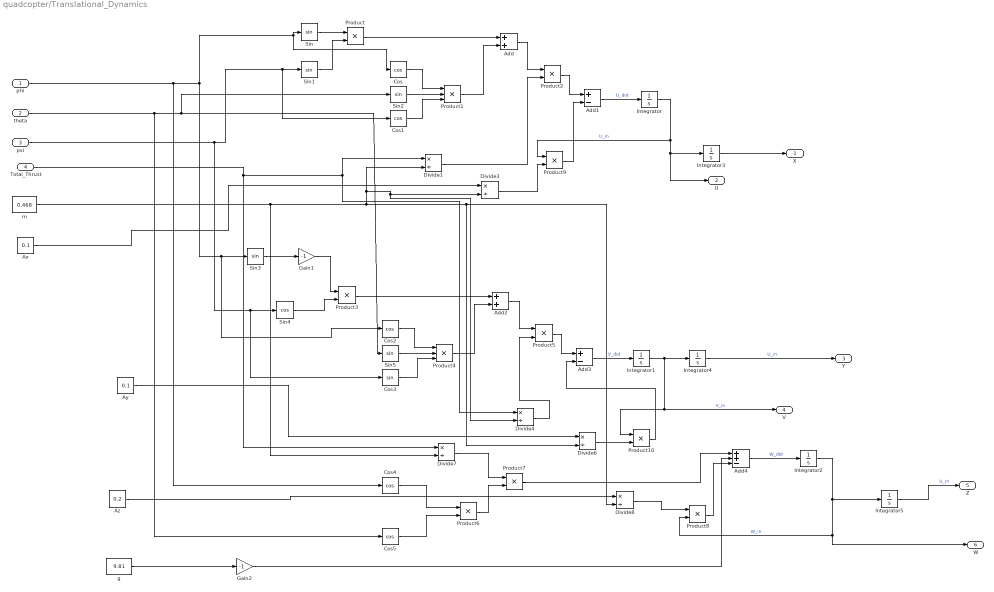
== system quadcopter/Translational_Dynamics ==
  phi : Inport
  theta : Inport  Port=2
  psi : Inport  Port=3
  Total_Thrust : Inport  Port=4
  Add : Sum
  Add1 : Sum  Inputs=+-
  Add2 : Sum
  Add3 : Sum  Inputs=+-
  Add4 : Sum  Inputs=++-
  Ax : Constant  Value=0.1
  Ay : Constant  Value=0.1
  Az : Constant  Value=0.2
  Cos{,1..2,4..5} (5 alike) : Trigonometry  Operator=cos
  Cos3 : Trigonometry
  Divide{1,3..4,6..8} (6 alike) : Product  Inputs=*/
  Gain1 : Gain  Gain=-1
  Gain2 : Gain  Gain=-1
  Integrator{,1..5} (6 alike) : Integrator
  Product{,2..3,5..10} (9 alike) : Product
  Product1 : Product  Inputs=3
  Product4 : Product  Inputs=3
  Sin{,1..3,5} (5 alike) : Trigonometry
  Sin4 : Trigonometry  Operator=cos
  g : Constant  Value=9.81
  m : Constant  Value=0.468
  X : Outport
  U : Outport  Port=2
  Y : Outport  Port=3
  V : Outport  Port=4
  Z : Outport  Port=5
  W : Outport  Port=6
  wires:
  Integrator1/1 -> Product10/1, V/1, Integrator4/1  "V_in"
  m/1 -> Divide7/2, Divide8/2, Divide6/2, Divide3/2, Divide4/2, Divide1/2
  Integrator2/1 -> Integrator5/1, W/1, Product8/2  "W_in"
  Product8/1 -> Add4/3
  Ay/1 -> Divide6/1
  Product2/1 -> Add1/1
  Integrator/1 -> Product9/1, U/1, Integrator3/1  "U_in"
  g/1 -> Gain2/1
  Product6/1 -> Product7/2
  phi/1 -> Cos2/1, Sin3/1, Sin/1, Cos/1, Cos4/1
  Integrator3/1 -> X/1
  Integrator5/1 -> Z/1  "U_in"
  Product7/1 -> Add4/1
  psi/1 -> Cos3/1, Sin4/1, Cos1/1, Sin1/1
  Product4/1 -> Add2/2
  Divide1/1 -> Product2/2
  Product9/1 -> Add1/2
  Divide7/1 -> Product7/1
  Sin/1 -> Product/1
  theta/1 -> Sin5/1, Sin2/1, Cos5/1
  Gain2/1 -> Add4/2
  Integrator4/1 -> Y/1  "U_in"
  Add/1 -> Product2/1
  Product1/1 -> Add/2
  Cos4/1 -> Product6/1
  Sin2/1 -> Product1/2
  Add1/1 -> Integrator/1  "U_dot"
  Total_Thrust/1 -> Divide7/1, Divide1/1, Divide4/1
  Cos/1 -> Product1/1
  Add3/1 -> Integrator1/1  "V_dot"
  Gain1/1 -> Product3/1
  Sin1/1 -> Product/2
  Add4/1 -> Integrator2/1  "W_dot"
  Cos5/1 -> Product6/2
  Product/1 -> Add/1
  Divide8/1 -> Product8/1
  Az/1 -> Divide8/1
  Divide3/1 -> Product9/2
  Sin5/1 -> Product4/2
  Cos1/1 -> Product1/3
  Ax/1 -> Divide3/1
  Cos3/1 -> Product4/3
  Product10/1 -> Add3/2
  Divide4/1 -> Product5/2
  Add2/1 -> Product5/1
  Sin4/1 -> Product3/2
  Sin3/1 -> Gain1/1
  Divide6/1 -> Product10/2
  Cos2/1 -> Product4/1
  Product3/1 -> Add2/1
  Product5/1 -> Add3/1

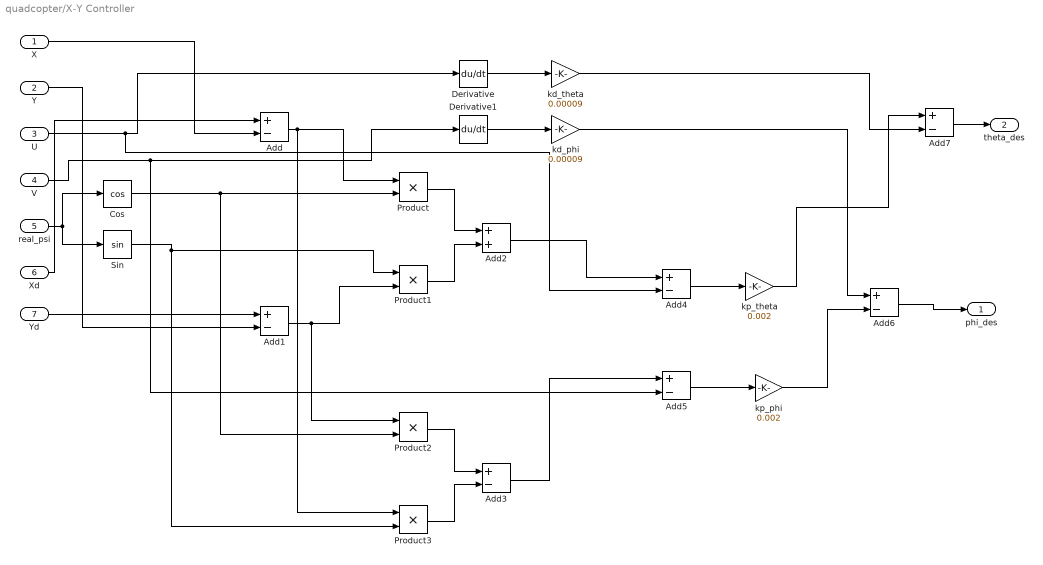
== system quadcopter/X-Y Controller ==
  X : Inport
  Y : Inport  Port=2
  U : Inport  Port=3
  V : Inport  Port=4
  real_psi : Inport  Port=5
  Xd : Inport  Port=6
  Yd : Inport  Port=7
  Add{,1,3..7} (7 alike) : Sum  Inputs=+-
  Add2 : Sum
  Cos : Trigonometry  Operator=cos
  Derivative : Derivative
  Derivative1 : Derivative
  Product{,1..3} (4 alike) : Product
  Sin : Trigonometry
  kd_phi : Gain  Gain=0.00009
  kd_theta : Gain  Gain=0.00009
  kp_phi : Gain  Gain=0.002
  kp_theta : Gain  Gain=0.002
  phi_des : Outport
  theta_des : Outport  Port=2
  wires:
  X/1 -> Add/2
  Xd/1 -> Add/1
  Yd/1 -> Add1/1
  Y/1 -> Add1/2
  real_psi/1 -> Sin/1, Cos/1
  Cos/1 -> Product2/2, Product/2
  Add/1 -> Product3/1, Product/1
  Add1/1 -> Product2/1, Product1/2
  Sin/1 -> Product1/1, Product3/2
  Product1/1 -> Add2/2
  Product/1 -> Add2/1
  Add2/1 -> Add4/1
  Product2/1 -> Add3/1
  Product3/1 -> Add3/2
  Add3/1 -> Add5/1
  U/1 -> Add4/2, Derivative/1
  V/1 -> Add5/2, Derivative1/1
  Derivative/1 -> kd_theta/1
  Derivative1/1 -> kd_phi/1
  Add4/1 -> kp_theta/1
  Add5/1 -> kp_phi/1
  kd_phi/1 -> Add6/1
  kp_phi/1 -> Add6/2
  kp_theta/1 -> Add7/1
  kd_theta/1 -> Add7/2
  Add6/1 -> phi_des/1
  Add7/1 -> theta_des/1

== matlab function quadcopter/sonsuzluk ==
  data: t input; ref_x output; ref_y output; ref_z output
function [ref_x, ref_y, ref_z] = fcn(t)
    % --- AYARLAR ---
    % Ölçek Katsayısı: Kalbin büyüklüğünü belirler.
    % 3 değeri ile Genişlik yakl. 48m, Uzunluk yakl. 50m olur (Eski A=50'ye denk)
    Scale = 1;       
    
    T_tur = 100;            % Bir tam kalp çizimi kaç saniye sürsün?
    
    Hedef_Yukseklik = 15;   % Çıkılacak son irtifa (metre)
    T_yukselme = 20;        % 15 metreye kaç saniyede çıksın?
    
    % --- HESAPLAMA ---
    % 0 ile 2*pi arasında değişen açı (Theta)
    theta = (2 * pi / T_tur) * t;
    
    % 1. X ve Y (Parametrik Kalp Formülü)
    % Orijinal Formül:
    % x = 16 * sin(theta)^3
    % y = 13*cos(theta) - 5*cos(2*theta) - 2*cos(3*theta) - cos(4*theta)
    
    % X Ekseni (Genişlik)
    ref_x = Scale * (16 * sin(theta)^3);
    
    % Y Ekseni (Uzunluk)
    % NOT: t=0 anında orijinal formül y=5 verir. 
    % Drone 0'dan başladığı için ani zıplama yapmasın diye -5 ile ofsetledik.
    y_ham = 13*cos(theta) - 5*cos(2*theta) - 2*cos(3*theta) - cos(4*theta);
    ref_y = Scale * (y_ham - 5); 
    
    % NOT: Eğer kalp ters duruyorsa veya yönü farklıysa:
    % ref_y = -1 * ref_y; % (Ters çevirmek için)
    % ref_x ve ref_y yer değiştirebilir (Yön değiştirmek için)
    
    % 2. Z (Yükselme Mantığı - Aynen Korundu)
    if t < T_yukselme
        % Rampa şeklinde yüksel
        ref_z = (Hedef_Yukseklik / T_yukselme) * t;
    else
        % İrtifayı koru
        ref_z = Hedef_Yukseklik;
    end
    
end

== matlab function quadcopter/MATLAB Function ==
  data: phi input; vrml_rot output; theta input; psi input
function vrml_rot = EulerToVRMLRot(phi, theta, psi)
% Bu fonksiyon, roll (phi), pitch (theta) ve yaw (psi) Euler açılarını
% VRML'nin beklediği Axis-Angle formatına dönüştürür.
% Girişler (radyan cinsinden):
% phi   : Roll açısı (X ekseni etrafında)
% theta : Pitch açısı (Y ekseni etrafında)
% psi   : Yaw açısı (Z ekseni etrafında)
% Çıkış (Axis-Angle formatında):
% vrml_rot = [eksen_x, eksen_y, eksen_z, açı_radyan]

% Genellikle MATLAB ve VRML arasındaki koordinat sistemi farklarını
% ve Euler açı sıra konvansiyonunu dikkate almak gerekir.
% Burada Z-Y-X (Yaw-Pitch-Roll) Euler dönüşüm sırasını kullanarak bir
% dönüşüm matrisi oluşturup, ardından bu matristen Axis-Angle'a dönüştüreceğiz.
% Simulink'teki VRML Viewer genellikle Z-Y-X konvansiyonunu iyi karşılar.

% Dönüşüm Matrisi Oluşturma (Z-Y-X Euler açısı sırası)
% R = Rz(psi) * Ry(theta) * Rx(phi)
Rx = [1 0 0; 0 cos(phi) -sin(phi); 0 sin(phi) cos(phi)];
Ry = [cos(theta) 0 sin(theta); 0 1 0; -sin(theta) 0 cos(theta)];
Rz = [cos(psi) -sin(psi) 0; sin(psi) cos(psi) 0; 0 0 1];

RotationMatrix = Rz * Ry * Rx;

% Dönüşüm Matrisinden Axis-Angle'a Dönüştürme
% (Bu dönüşüm için temel bir algoritma kullanılmıştır)
traceR = RotationMatrix(1,1) + RotationMatrix(2,2) + RotationMatrix(3,3);
angle = acos((traceR - 1) / 2);

if abs(angle) < 1e-6 % Açı çok küçükse veya sıfırsa
    axis = [0 0 1]; % Herhangi bir eksen olabilir, Z varsayalım
    angle = 0;
elseif abs(angle - pi) < 1e-6 % Açı 180 derece ise
    % Bu durum için daha dikkatli hesaplama gerekir,
    % örneğin sütunlar arası farklardan eksen bulunur.
    % Şimdilik bu durumu basitleştirelim veya varsayalım ki nadir olacak.
    % Daha sağlam bir yaklaşım için https://www.euclideanspace.com/maths/geometry/rotations/conversions/matrixToAngle/index.htm
    % gibi kaynaklara başvurulabilir.
    % Basit bir 180 derece dönüş ekseni bulma:
    axis_x = RotationMatrix(1,1) + 1;
    axis_y = RotationMatrix(2,2) + 1;
    axis_z = RotationMatrix(3,3) + 1;
    % En büyük bileşeni bulup normalize et
    max_val = max([axis_x, axis_y, axis_z]);
    if max_val == 0
        axis = [1 0 0]; % Varsayılan
    else
        axis = [axis_x, axis_y, axis_z] / max_val; % Normalizasyon sadece yönü korur.
    end
else
    % Normal durum
    axis_x = RotationMatrix(3,2) - RotationMatrix(2,3);
    axis_y = RotationMatrix(1,3) - RotationMatrix(3,1);
    axis_z = RotationMatrix(2,1) - RotationMatrix(1,2);
    axis_magnitude = norm([axis_x, axis_y, axis_z]);

    if axis_magnitude < 1e-6 % Neredeyse sıfır dönme
        axis = [0 0 1]; % Varsayılan
        angle = 0;
    else
        axis = [axis_x, axis_y, axis_z] / axis_magnitude;
    end
end

vrml_rot = [axis(1); axis(2); axis(3); angle];

end

== matlab function quadcopter/spiral1 ==
  data: t input; ref_x output; ref_y output; ref_z output
function [ref_x, ref_y, ref_z] = fcn(t)
    % --- AYARLAR ---
    R = 5;          % Yarıçap (Sabit 5 metre)
    T_tur = 150;     % Bir tam turu kaç saniyede atsın?
    V_z = 0.5;      % Saniyede kaç metre yükselsin?
    
    % --- HESAPLAMA ---
    w = (2 * pi) / T_tur; % Açısal hız
    
    % Çember Denklemi (Sabit R ile)
    % t=0 anında (R, 0) noktasından başlar
    ref_x = R * cos(w * t); 
    ref_y = R * sin(w * t);
    
    % Yükseklik (Zamanla artar)
    ref_z = V_z * t;
end
